simulink model "TST_EngDa_TEng"  (R2016b)
settings: Solver=FixedStepDiscrete  StartTime=0.0  StopTime=0.4  FixedStep=sampleTime  RelTol=1e-3
values from neighbouring files (symbols this model uses):
  testCase = 1    [initTST_EngDa_TEng_001.m]
libraries: simulink x6, UnitTest_Lib x4
settings Model: Creator=caijinkang  LastModifiedBy=caijinkang
settings DebuggingCC: SignalRangeChecking=error

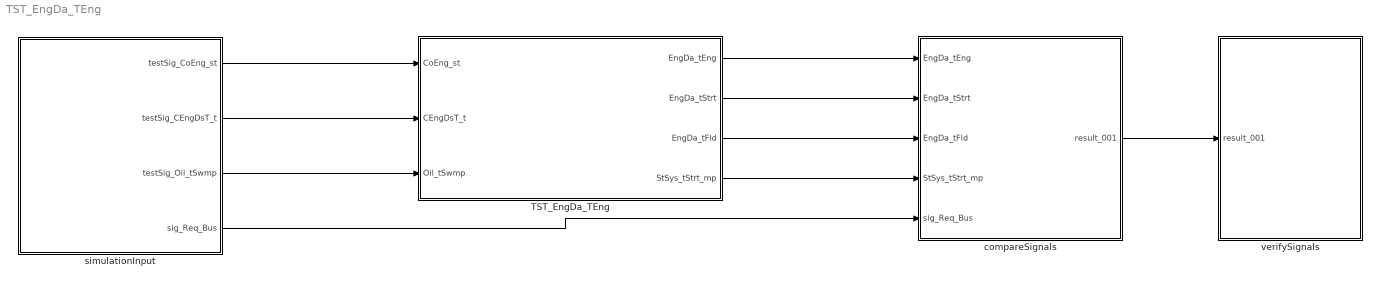
== system TST_EngDa_TEng ==
  TST_EngDa_TEng : Subsystem
  compareSignals : Subsystem
  simulationInput : Subsystem
  verifySignals : Subsystem
  wires:
  simulationInput/1(testSig_CoEng_st) -> TST_EngDa_TEng/1(CoEng_st)
  simulationInput/2(testSig_CEngDsT_t) -> TST_EngDa_TEng/2(CEngDsT_t)
  simulationInput/3(testSig_Oil_tSwmp) -> TST_EngDa_TEng/3(Oil_tSwmp)
  TST_EngDa_TEng/1(EngDa_tEng) -> compareSignals/1(EngDa_tEng)
  TST_EngDa_TEng/2(EngDa_tStrt) -> compareSignals/2(EngDa_tStrt)
  TST_EngDa_TEng/3(EngDa_tFld) -> compareSignals/3(EngDa_tFld)
  TST_EngDa_TEng/4(StSys_tStrt_mp) -> compareSignals/4(StSys_tStrt_mp)
  simulationInput/4(sig_Req_Bus) -> compareSignals/5(sig_Req_Bus)
  compareSignals/1(result_001) -> verifySignals/1(result_001)

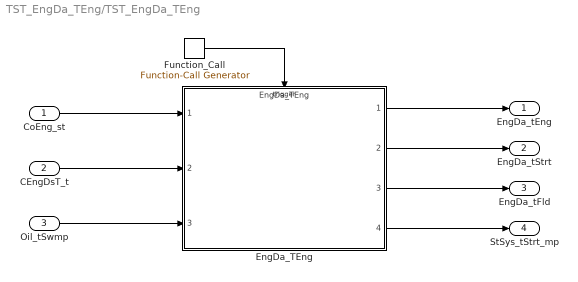
== system TST_EngDa_TEng/TST_EngDa_TEng ==
  CoEng_st : Inport
  CEngDsT_t : Inport  Port=2
  Oil_tSwmp : Inport  Port=3
  EngDa_TEng : ModelReference  ModelNameDialog=EngDa_TEng  SimulationMode=Normal  ModelReferenceVersion=1.11  TriggerPortName=function  TriggerPortTriggerType=function-call  TriggerPortStatesWhenEnabling=held
  Function_Call : simulink/Ports & Subsystems/Function-Call Generator  sample_time=sampleTime  numberOfIterations=1
  EngDa_tEng : Outport
  EngDa_tStrt : Outport  Port=2
  EngDa_tFld : Outport  Port=3
  StSys_tStrt_mp : Outport  Port=4
  wires:
  Function_Call/1 -> EngDa_TEng/Trigger
  CoEng_st/1 -> EngDa_TEng/1
  CEngDsT_t/1 -> EngDa_TEng/2
  Oil_tSwmp/1 -> EngDa_TEng/3
  EngDa_TEng/1 -> EngDa_tEng/1
  EngDa_TEng/2 -> EngDa_tStrt/1
  EngDa_TEng/3 -> EngDa_tFld/1
  EngDa_TEng/4 -> StSys_tStrt_mp/1

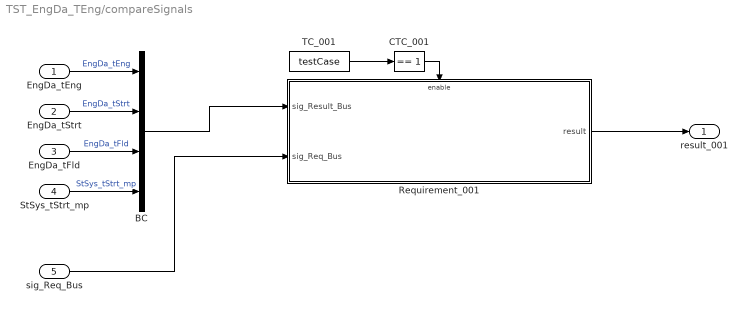
== system TST_EngDa_TEng/compareSignals ==
  EngDa_tEng : Inport
  EngDa_tStrt : Inport  Port=2
  EngDa_tFld : Inport  Port=3
  StSys_tStrt_mp : Inport  Port=4
  sig_Req_Bus : Inport  Port=5
  BC : BusCreator  Inputs=4
  CTC_001 : simulink/Logic and Bit Operations/Compare To Constant  relop===  const=1  OutDataTypeStr=boolean
  Requirement_001 : Subsystem
  TC_001 : Constant  Value=testCase
  result_001 : Outport
  wires:
  EngDa_tEng/1 -> BC/1  "EngDa_tEng"
  EngDa_tStrt/1 -> BC/2  "EngDa_tStrt"
  EngDa_tFld/1 -> BC/3  "EngDa_tFld"
  StSys_tStrt_mp/1 -> BC/4  "StSys_tStrt_mp"
  TC_001/1 -> CTC_001/1
  CTC_001/1 -> Requirement_001/Enable
  sig_Req_Bus/1 -> Requirement_001/2(sig_Req_Bus)
  BC/1 -> Requirement_001/1(sig_Result_Bus)
  Requirement_001/1(result) -> result_001/1

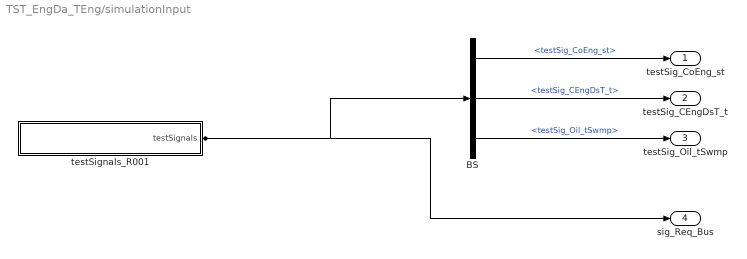
== system TST_EngDa_TEng/simulationInput ==
  BS : BusSelector  OutputSignals=testSig_CoEng_st,testSig_CEngDsT_t,testSig_Oil_tSwmp
  testSignals_R001 : Subsystem
  testSig_CoEng_st : Outport
  testSig_CEngDsT_t : Outport  Port=2
  testSig_Oil_tSwmp : Outport  Port=3
  sig_Req_Bus : Outport  Port=4
  wires:
  BS/1 -> testSig_CoEng_st/1  "<testSig_CoEng_st>"
  BS/2 -> testSig_CEngDsT_t/1  "<testSig_CEngDsT_t>"
  BS/3 -> testSig_Oil_tSwmp/1  "<testSig_Oil_tSwmp>"
  testSignals_R001/1(testSignals) -> BS/1, sig_Req_Bus/1

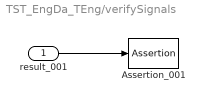
== system TST_EngDa_TEng/verifySignals ==
  result_001 : Inport
  Assertion_001 : Assertion
  wires:
  result_001/1 -> Assertion_001/1

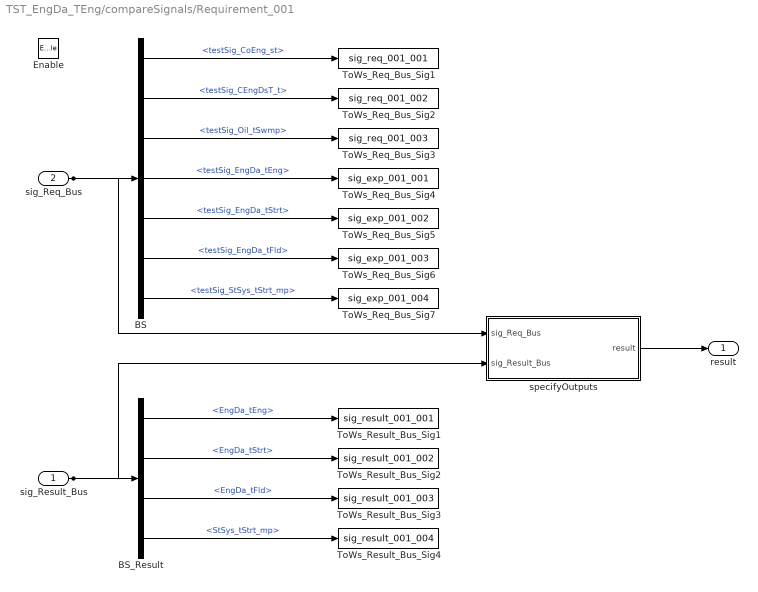
== system TST_EngDa_TEng/compareSignals/Requirement_001 ==
  sig_Result_Bus : Inport
  sig_Req_Bus : Inport  Port=2
  Enable : EnablePort
  BS : BusSelector  OutputSignals=testSig_CoEng_st,testSig_CEngDsT_t,testSig_Oil_tSwmp,testSig_EngDa_tEng,testSig_EngDa_tStrt,testSig_EngDa_tFld,testSig_StSys_tStrt_mp
  BS_Result : BusSelector  OutputSignals=EngDa_tEng,EngDa_tStrt,EngDa_tFld,StSys_tStrt_mp
  ToWs_Req_Bus_Sig1 : ToWorkspace  VariableName=sig_req_001_001  SaveFormat=Structure With Time
  ToWs_Req_Bus_Sig2 : ToWorkspace  VariableName=sig_req_001_002  SaveFormat=Structure With Time
  ToWs_Req_Bus_Sig3 : ToWorkspace  VariableName=sig_req_001_003  SaveFormat=Structure With Time
  ToWs_Req_Bus_Sig4 : ToWorkspace  VariableName=sig_exp_001_001  SaveFormat=Structure With Time
  ToWs_Req_Bus_Sig5 : ToWorkspace  VariableName=sig_exp_001_002  SaveFormat=Structure With Time
  ToWs_Req_Bus_Sig6 : ToWorkspace  VariableName=sig_exp_001_003  SaveFormat=Structure With Time
  ToWs_Req_Bus_Sig7 : ToWorkspace  VariableName=sig_exp_001_004  SaveFormat=Structure With Time
  ToWs_Result_Bus_Sig1 : ToWorkspace  VariableName=sig_result_001_001  SaveFormat=Structure With Time
  ToWs_Result_Bus_Sig2 : ToWorkspace  VariableName=sig_result_001_002  SaveFormat=Structure With Time
  ToWs_Result_Bus_Sig3 : ToWorkspace  VariableName=sig_result_001_003  SaveFormat=Structure With Time
  ToWs_Result_Bus_Sig4 : ToWorkspace  VariableName=sig_result_001_004  SaveFormat=Structure With Time
  specifyOutputs : Subsystem
  result : Outport
  wires:
  sig_Req_Bus/1 -> BS/1, specifyOutputs/1(sig_Req_Bus)
  BS/1 -> ToWs_Req_Bus_Sig1/1  "<testSig_CoEng_st>"
  BS/2 -> ToWs_Req_Bus_Sig2/1  "<testSig_CEngDsT_t>"
  BS/3 -> ToWs_Req_Bus_Sig3/1  "<testSig_Oil_tSwmp>"
  BS/4 -> ToWs_Req_Bus_Sig4/1  "<testSig_EngDa_tEng>"
  BS/5 -> ToWs_Req_Bus_Sig5/1  "<testSig_EngDa_tStrt>"
  BS/6 -> ToWs_Req_Bus_Sig6/1  "<testSig_EngDa_tFld>"
  BS/7 -> ToWs_Req_Bus_Sig7/1  "<testSig_StSys_tStrt_mp>"
  sig_Result_Bus/1 -> BS_Result/1, specifyOutputs/2(sig_Result_Bus)
  BS_Result/1 -> ToWs_Result_Bus_Sig1/1  "<EngDa_tEng>"
  BS_Result/2 -> ToWs_Result_Bus_Sig2/1  "<EngDa_tStrt>"
  BS_Result/3 -> ToWs_Result_Bus_Sig3/1  "<EngDa_tFld>"
  BS_Result/4 -> ToWs_Result_Bus_Sig4/1  "<StSys_tStrt_mp>"
  specifyOutputs/1(result) -> result/1

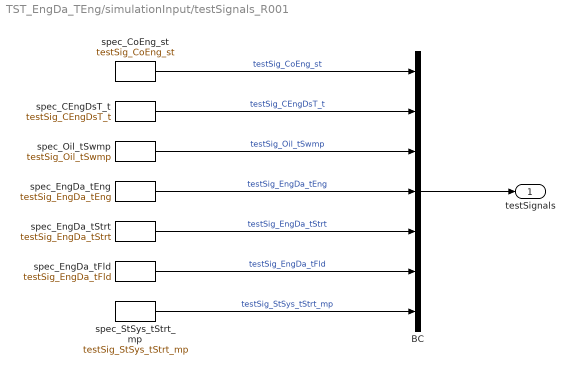
== system TST_EngDa_TEng/simulationInput/testSignals_R001 ==
  BC : BusCreator  Inputs=7
  spec_CEngDsT_t : FromWorkspace  VariableName=testSig_CEngDsT_t  Interpolate=off  OutputAfterFinalValue=Holding final value
  spec_CoEng_st : FromWorkspace  VariableName=testSig_CoEng_st  Interpolate=off  OutputAfterFinalValue=Holding final value
  spec_EngDa_tEng : FromWorkspace  VariableName=testSig_EngDa_tEng  Interpolate=off  OutputAfterFinalValue=Holding final value
  spec_EngDa_tFld : FromWorkspace  VariableName=testSig_EngDa_tFld  Interpolate=off  OutputAfterFinalValue=Holding final value
  spec_EngDa_tStrt : FromWorkspace  VariableName=testSig_EngDa_tStrt  Interpolate=off  OutputAfterFinalValue=Holding final value
  spec_Oil_tSwmp : FromWorkspace  VariableName=testSig_Oil_tSwmp  Interpolate=off  OutputAfterFinalValue=Holding final value
  spec_StSys_tStrt_mp : FromWorkspace  VariableName=testSig_StSys_tStrt_mp  Interpolate=off  OutputAfterFinalValue=Holding final value
  testSignals : Outport
  wires:
  BC/1 -> testSignals/1
  spec_CoEng_st/1 -> BC/1  "testSig_CoEng_st"
  spec_CEngDsT_t/1 -> BC/2  "testSig_CEngDsT_t"
  spec_Oil_tSwmp/1 -> BC/3  "testSig_Oil_tSwmp"
  spec_EngDa_tEng/1 -> BC/4  "testSig_EngDa_tEng"
  spec_EngDa_tStrt/1 -> BC/5  "testSig_EngDa_tStrt"
  spec_EngDa_tFld/1 -> BC/6  "testSig_EngDa_tFld"
  spec_StSys_tStrt_mp/1 -> BC/7  "testSig_StSys_tStrt_mp"

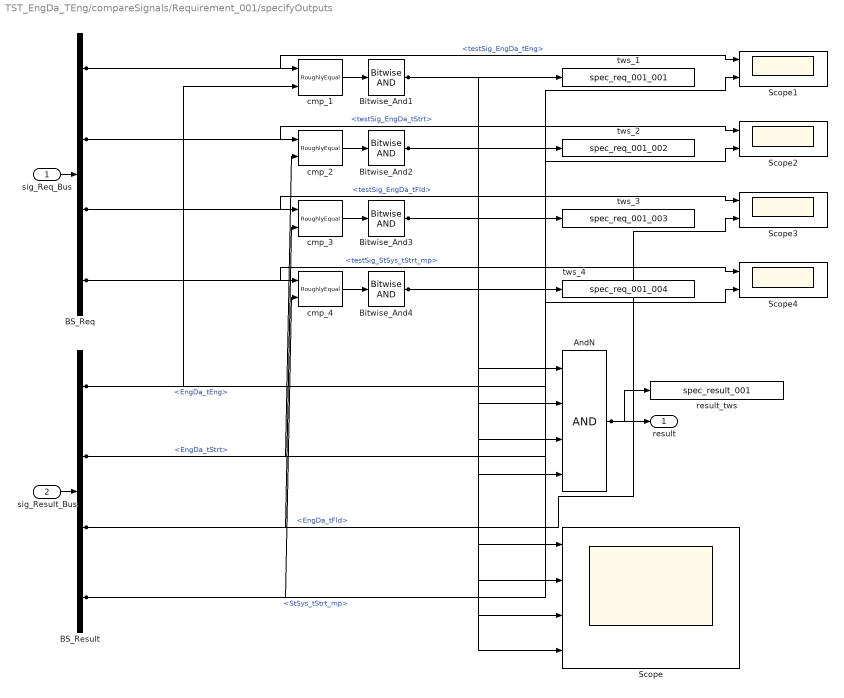
== system TST_EngDa_TEng/compareSignals/Requirement_001/specifyOutputs ==
  sig_Req_Bus : Inport
  sig_Result_Bus : Inport  Port=2
  AndN : Logic  Inputs=4
  BS_Req : BusSelector  OutputSignals=testSig_EngDa_tEng,testSig_EngDa_tStrt,testSig_EngDa_tFld,testSig_StSys_tStrt_mp
  BS_Result : BusSelector  OutputSignals=EngDa_tEng,EngDa_tStrt,EngDa_tFld,StSys_tStrt_mp
  Bitwise_And{1..4} (4 alike) : simulink/Logic and Bit Operations/Bitwise Operator  logicop=AND  UseBitMask=off  BitMask=bin2dec('11011001')  BitMaskRealWorld=Stored Integer
  Scope : Scope  NumInputPorts=4
  Scope{1..4} (4 alike) : Scope  NumInputPorts=2
  cmp_{1..4} (4 alike) : UnitTest_Lib/RoughlyEqual  slope=0.1
  result_tws : ToWorkspace  VariableName=spec_result_001
  tws_1 : ToWorkspace  VariableName=spec_req_001_001
  tws_2 : ToWorkspace  VariableName=spec_req_001_002
  tws_3 : ToWorkspace  VariableName=spec_req_001_003
  tws_4 : ToWorkspace  VariableName=spec_req_001_004
  result : Outport
  wires:
  sig_Req_Bus/1 -> BS_Req/1
  sig_Result_Bus/1 -> BS_Result/1
  AndN/1 -> result/1, result_tws/1
  BS_Req/1 -> cmp_1/1, Scope1/1  "<testSig_EngDa_tEng>"
  BS_Result/1 -> cmp_1/2, Scope1/2  "<EngDa_tEng>"
  cmp_1/1 -> Bitwise_And1/1
  Bitwise_And1/1 -> tws_1/1, AndN/1, Scope/1
  BS_Req/2 -> cmp_2/1, Scope2/1  "<testSig_EngDa_tStrt>"
  BS_Result/2 -> cmp_2/2, Scope2/2  "<EngDa_tStrt>"
  cmp_2/1 -> Bitwise_And2/1
  Bitwise_And2/1 -> tws_2/1, AndN/2, Scope/2
  BS_Req/3 -> cmp_3/1, Scope3/1  "<testSig_EngDa_tFld>"
  BS_Result/3 -> cmp_3/2, Scope3/2  "<EngDa_tFld>"
  cmp_3/1 -> Bitwise_And3/1
  Bitwise_And3/1 -> tws_3/1, AndN/3, Scope/3
  BS_Req/4 -> cmp_4/1, Scope4/1  "<testSig_StSys_tStrt_mp>"
  BS_Result/4 -> cmp_4/2, Scope4/2  "<StSys_tStrt_mp>"
  cmp_4/1 -> Bitwise_And4/1
  Bitwise_And4/1 -> tws_4/1, AndN/4, Scope/4
